simulink model "SMC_2DOF2018a"  (R2018a)
settings: Solver=FixedStepAuto  StartTime=0.0  StopTime=5  FixedStep=0.01  RelTol=1e-3
libraries: simulink x2
settings Model: Creator=htb  LastModifiedBy=htb
settings DataIOCC: ReturnWorkspaceOutputs=on
settings SFSimCC: SimUseLocalCustomCode=on
settings RTWCC: RTWUseLocalCustomCode=on

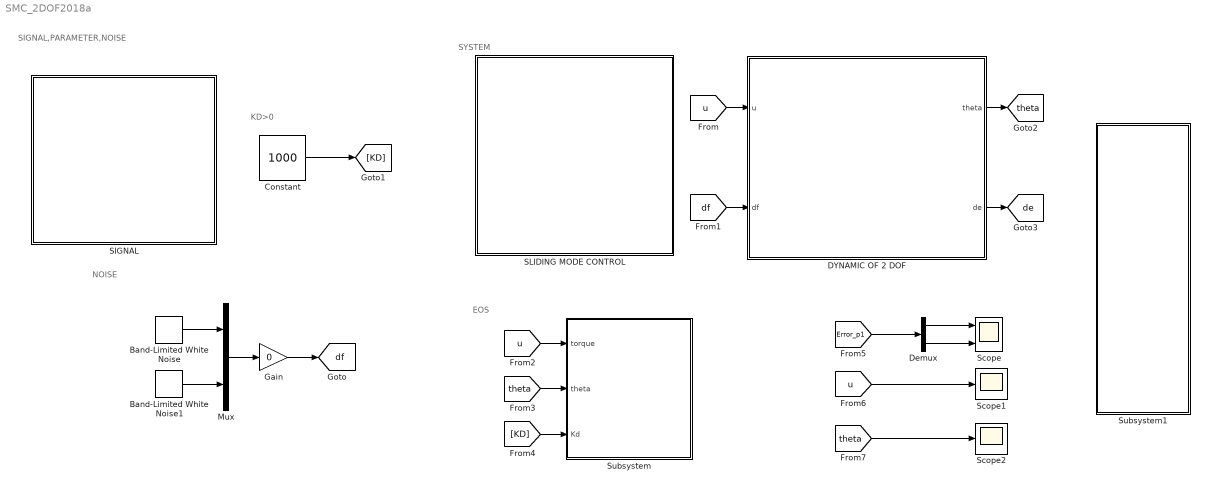
== system SMC_2DOF2018a ==
  note: EOS
  note: SYSTEM
  note: SIGNAL,PARAMETER,NOISE
  note: KD>0
  note: NOISE
  Band-Limited White Noise : simulink/Sources/Band-Limited White Noise  Cov=[0.003]  Ts=0.01  seed=[23341]
  Band-Limited White Noise1 : simulink/Sources/Band-Limited White Noise  Cov=[0.003]  Ts=0.01  seed=[23341]
  Constant : Constant  Value=1000
  DYNAMIC OF 2 DOF : Subsystem
  Demux : Demux  Outputs=2
  Gain : Gain  Gain=0
  Mux : Mux  Inputs=2
  SIGNAL : Subsystem
  SLIDING MODE CONTROL : Subsystem
  Scope : Scope  NumInputPorts=2
  Scope1 : Scope
  Scope2 : Scope
  Subsystem : Subsystem
  Subsystem1 : Subsystem
  tag scope: de=global, df=global, theta=global
  wires:
  Mux/1 -> Gain/1
  Band-Limited White Noise/1 -> Mux/1
  Band-Limited White Noise1/1 -> Mux/2
  Gain/1 -> [df]
  Constant/1 -> [KD]
  [u] -> DYNAMIC OF 2 DOF/1(u)
  [df] -> DYNAMIC OF 2 DOF/2(df)
  DYNAMIC OF 2 DOF/1(theta) -> [theta]
  [u] -> Subsystem/1("torque ")
  [theta] -> Subsystem/2(theta)
  [KD] -> Subsystem/3(Kd)
  DYNAMIC OF 2 DOF/2(de) -> [de]
  Demux/1 -> Scope/1
  Demux/2 -> Scope/2
  [Error_p1] -> Demux/1
  [u] -> Scope1/1
  [theta] -> Scope2/1

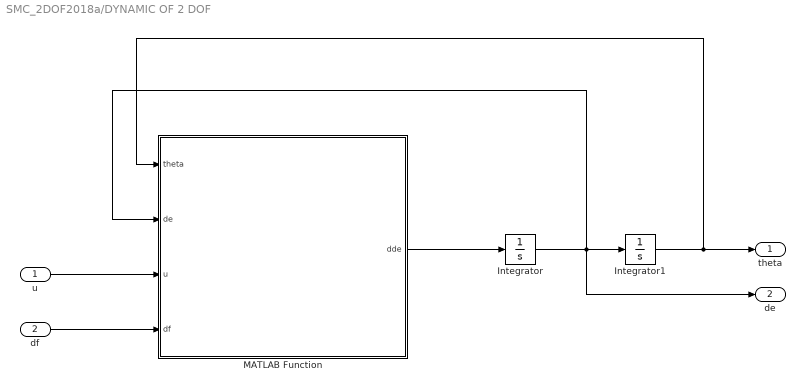
== system SMC_2DOF2018a/DYNAMIC OF 2 DOF ==
  u : Inport
  df : Inport  Port=2
  Integrator : Integrator  InitialCondition=zeros(2,1)
  Integrator1 : Integrator  InitialCondition=zeros(2,1)
  MATLAB Function : MATLAB Function  TreatAsAtomicUnit=on
  theta : Outport
  de : Outport  Port=2
  wires:
  u/1 -> MATLAB Function/3(u)
  df/1 -> MATLAB Function/4(df)
  MATLAB Function/1(dde) -> Integrator/1
  Integrator/1 -> MATLAB Function/2(de), de/1, Integrator1/1
  Integrator1/1 -> MATLAB Function/1(theta), theta/1

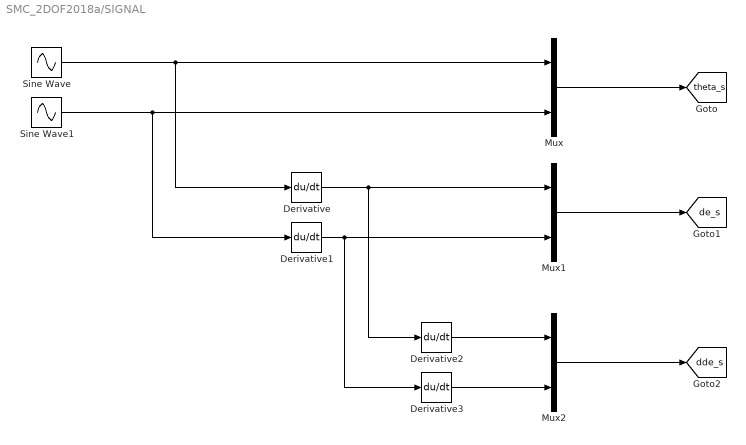
== system SMC_2DOF2018a/SIGNAL ==
  Derivative{,1..3} (4 alike) : Derivative
  Mux : Mux  Inputs=2
  Mux1 : Mux  Inputs=2
  Mux2 : Mux  Inputs=2
  Sine Wave : Sin  Amplitude=pi/3  Frequency=2*pi/3  SampleTime=0
  Sine Wave1 : Sin  Amplitude=pi/6  Frequency=2*pi/3  SampleTime=0
  tag scope: dde_s=global, de_s=global, theta_s=global
  wires:
  Sine Wave/1 -> Derivative/1, Mux/1
  Sine Wave1/1 -> Derivative1/1, Mux/2
  Mux/1 -> [theta_s]
  Mux1/1 -> [de_s]
  Derivative/1 -> Derivative2/1, Mux1/1
  Derivative1/1 -> Derivative3/1, Mux1/2
  Derivative2/1 -> Mux2/1
  Derivative3/1 -> Mux2/2
  Mux2/1 -> [dde_s]

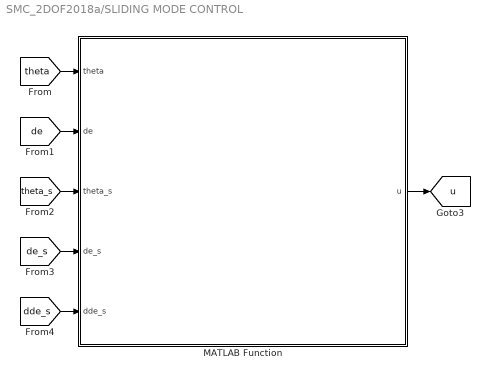
== system SMC_2DOF2018a/SLIDING MODE CONTROL ==
  MATLAB Function : MATLAB Function  TreatAsAtomicUnit=on
  tag scope: u=global
  wires:
  [de] -> MATLAB Function/2(de)
  MATLAB Function/1(u) -> [u]
  [dde_s] -> MATLAB Function/5(dde_s)
  [theta] -> MATLAB Function/1(theta)
  [de_s] -> MATLAB Function/4(de_s)
  [theta_s] -> MATLAB Function/3(theta_s)

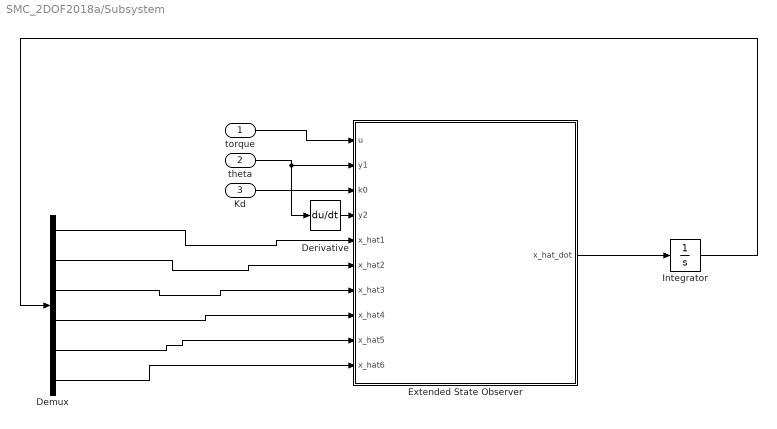
== system SMC_2DOF2018a/Subsystem ==
  "torque " : Inport
  theta : Inport  Port=2
  Kd : Inport  Port=3
  Demux : Demux  Outputs=6
  Derivative : Derivative
  Extended State Observer : MATLAB Function  TreatAsAtomicUnit=on
  Integrator : Integrator  InitialCondition=[]
  wires:
  Extended State Observer/1(x_hat_dot) -> Integrator/1
  Demux/1 -> Extended State Observer/5(x_hat1)
  Demux/2 -> Extended State Observer/6(x_hat2)
  Demux/3 -> Extended State Observer/7(x_hat3)
  Demux/4 -> Extended State Observer/8(x_hat4)
  Demux/5 -> Extended State Observer/9(x_hat5)
  Demux/6 -> Extended State Observer/10(x_hat6)
  Integrator/1 -> Demux/1
  "torque "/1 -> Extended State Observer/1(u)
  theta/1 -> Derivative/1, Extended State Observer/2(y1)
  Kd/1 -> Extended State Observer/3(k0)
  Derivative/1 -> Extended State Observer/4(y2)

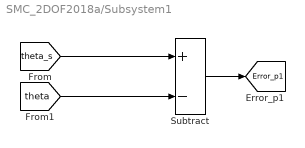
== system SMC_2DOF2018a/Subsystem1 ==
  Subtract : Sum  Inputs=+-
  tag scope: Error_p1=global
  wires:
  [theta_s] -> Subtract/1
  [theta] -> Subtract/2
  Subtract/1 -> [Error_p1]

== matlab function SMC_2DOF2018a/DYNAMIC OF 2 DOF/MATLAB Function ==
  data: theta input; de input; u input; dde output; df input
function dde = DYN_2DOF(theta,de,u,df)
%% decalre parameter
m1 = 0.17;
m2 = 0.09;
L1 = 0.09;
L2 = 0.12;
I1 = -3.788963153993949e-04;
I2 = 8.783917785597624e-05;
x1 = 0.043780593805964;
x2 = 0.056187713639820;
y1 = 0;
y2 = 0;
z1 = 0;
z2 = 0;
g = 9.81;
% syms theta1 theta2 de1 de2 dde1 dde2 
t1 = theta(1);
t2 = theta(2);
dt1 = de(1);
dt2 = de(2);
%% M 
M = [ (9*L1^2)/100 + (9*cos(t2)*L1*x2)/50 - (9*sin(t2)*L1*y2)/50 + (17*x1^2)/100 + (9*x2^2)/100 + (17*y1^2)/100 + (9*y2^2)/100 - 1342264131772481/4611686018427387904, (9*x2^2)/100 + (9*L1*cos(t2)*x2)/100 + (9*y2^2)/100 - (9*L1*sin(t2)*y2)/100 + 1620346833554249/18446744073709551616;
                                             (9*x2^2)/100 + (9*L1*cos(t2)*x2)/100 + (9*y2^2)/100 - (9*L1*sin(t2)*y2)/100 + 1620346833554249/18446744073709551616,                                                         (9*x2^2)/100 + (9*y2^2)/100 + 1620346833554249/18446744073709551616]
                                      
%% C
C =[           -(9*L1*dt2*(y2*cos(t2) + x2*sin(t2)))/50, -(9*L1*dt2*(y2*cos(t2) + x2*sin(t2)))/100;
     (9*L1*(y2*cos(t2) + x2*sin(t2))*(2*dt1 - dt2))/200,  (9*L1*dt1*(y2*cos(t2) + x2*sin(t2)))/200]

%% G
G =[ - (17*g*(x1*cos(t1) - y1*sin(t1)))/100 - (9*g*(x2*cos(t1 + t2) + L1*cos(t1) - y2*sin(t1 + t2)))/100;
                                                                  -(9*g*(x2*cos(t1 + t2) - y2*sin(t1 + t2)))/100]
                                                              

%% dde                                                              
dde = inv(M)*u + inv(M)*(-C*de - G) - inv(M)*df;

== matlab function SMC_2DOF2018a/SLIDING MODE CONTROL/MATLAB Function ==
  data: theta input; u output; de input; theta_s input; de_s input; dde_s input
function u = SMC(theta,de,theta_s,de_s,dde_s)

%% decalre parameter
m1 = 0.17;
m2 = 0.09;
L1 = 0.09;
L2 = 0.12;
I1 = -3.788963153993949e-04;
I2 = 8.783917785597624e-05;
x1 = 0.043780593805964;
x2 = 0.056187713639820;
y1 = 0;
y2 = 0;
z1 = 0;
z2 = 0;
g = 9.81;
% syms theta1 theta2 de1 de2 dde1 dde2 
t1 = theta(1);
t2 = theta(2);
dt1 = de(1);
dt2 = de(2);
%% M 
M = [ (9*L1^2)/100 + (9*cos(t2)*L1*x2)/50 - (9*sin(t2)*L1*y2)/50 + (17*x1^2)/100 + (9*x2^2)/100 + (17*y1^2)/100 + (9*y2^2)/100 - 1342264131772481/4611686018427387904, (9*x2^2)/100 + (9*L1*cos(t2)*x2)/100 + (9*y2^2)/100 - (9*L1*sin(t2)*y2)/100 + 1620346833554249/18446744073709551616;
                                             (9*x2^2)/100 + (9*L1*cos(t2)*x2)/100 + (9*y2^2)/100 - (9*L1*sin(t2)*y2)/100 + 1620346833554249/18446744073709551616,                                                         (9*x2^2)/100 + (9*y2^2)/100 + 1620346833554249/18446744073709551616]
                                      
%% C
C =[           -(9*L1*dt2*(y2*cos(t2) + x2*sin(t2)))/50, -(9*L1*dt2*(y2*cos(t2) + x2*sin(t2)))/100;
     (9*L1*(y2*cos(t2) + x2*sin(t2))*(2*dt1 - dt2))/200,  (9*L1*dt1*(y2*cos(t2) + x2*sin(t2)))/200]

%% G
G =[ - (17*g*(x1*cos(t1) - y1*sin(t1)))/100 - (9*g*(x2*cos(t1 + t2) + L1*cos(t1) - y2*sin(t1 + t2)))/100;
                                                                  -(9*g*(x2*cos(t1 + t2) - y2*sin(t1 + t2)))/100]
                                                              


%% sliding mode control
lamda = [20 0 ; 0 20];
k = [1 0 ;0 1]; 
k1 = [40 0 ;0 40];

e1 = theta - theta_s;
e2 = de - de_s;
s = lamda*e1 + e2;
u = M*(dde_s - lamda*e2 - k1*s - k*sign(s) + C*(de_s-lamda*e1) + G)

== matlab function SMC_2DOF2018a/Subsystem/Extended State Observer ==
  data: x_hat_dot output; u input; y1 input; k0 input; y2 input; x_hat1 input; x_hat2 input; x_hat3 input; x_hat4 input; x_hat5 input; x_hat6 input
function x_hat_dot  = EOS(u,y1,k0,y2,x_hat1,x_hat2,x_hat3,x_hat4,x_hat5,x_hat6)
%% MGV
t1 = y1(1);
t2 = y1(2);
dt1 = y2(1);
dt2 = y2(2);

M = [  (40993608526197147*cos(t2))/45035996273704960000 + 2416348354571775/2305843009213693952, (40993608526197147*cos(t2))/90071992547409920000 + 6861718451819221/18446744073709551616;...
(40993608526197147*cos(t2))/90071992547409920000 + 6861718451819221/18446744073709551616,                                                        6861718451819221/18446744073709551616];
 
 
C = [           -(40993608526197147*dt2*sin(t2))/45035996273704960000, -(40993608526197147*dt2*sin(t2))/90071992547409920000;...
(40993608526197147*sin(t2)*(2*dt1 - dt2))/180143985094819840000, (40993608526197147*dt1*sin(t2))/180143985094819840000];
 
 
G = [- (4468303329355489023*cos(t1 + t2))/90071992547409920000 - (5493451060130401225773*cos(t1))/36028797018963968000000;...
                                                                 -(4468303329355489023*cos(t1 + t2))/90071992547409920000];
 

  %% matrix
  x1_hat = [x_hat1;x_hat2]; %theta
  x2_hat = [x_hat3;x_hat4]; %theta_d
  x3_hat = [x_hat5;x_hat6]; %noise
  H = inv(M);
  F = -H * (C * x2_hat + G);
  An = [0 0 1 0 0 0;...
        0 0 0 1 0 0;...
        0 0 0 0 1 0;...
        0 0 0 0 0 1;...
        0 0 0 0 0 0;...
        0 0 0 0 0 0];
  Bn = [0 0;...
        0 0;...
        H(1,1) H(1,2);...
        H(2,1) H(2,2);...
        0 0;...
        0 0];
  x_hat = [x_hat1;...
           x_hat2;...
           x_hat3;...
           x_hat4;...
           x_hat5;...
           x_hat6];
       
  phi_x_hat = [0;...
               0;...
               F(1,1);...
               F(2,1);...
               0;...
               0];
      
  K = [3*k0 0;...
       0    3*k0;...
       3*k0^2   0;...
       0    3*k0^2;...
       k0^3 0;...
       0    k0^3];
 
 %% the EOS 
 x_hat_dot = An*x_hat +Bn*u + phi_x_hat + K*(y1 - x1_hat);
%  denta = [2,1;1,2] * x3_hat;
